simulink model "WaterTankSysControl2024"  (R2024a)
settings: Solver=FixedStepAuto  StartTime=0.0  StopTime=525  FixedStep=0.75  RelTol=1e-3  EnableMultiTasking=on
StopFcn:
  | FileName='SFControlData0.mat';
  | [fPath, fName, fExt] = fileparts(FileName);
  | if isempty(fExt)  % No '.mat' in FileName
  |     fExt     = '.mat';
  |     FileName = fullfile(fPath, [fName, fExt]);
  | end
  | if exist(FileName, 'file')
  |     % Get number of files:
  |     fDir     = dir(fullfile(fPath, [fName, '*', fExt]));
  |     fStr     = lower(sprintf('%s*', fDir.name));
  |     %fNum     = sscanf(fStr, [fName, '%d', fExt, '*']);
  |     digit =  str2double(extract(fStr, digitsPattern));
  |     %newNum = digit + 1;
  |     if isempty(digit)
  |         newNum = 1;
  |     else
  |         newNum = digit + 1;
  |     end
  |     FileName = fullfile(fPath, [fName, sprintf('%d', newNum(end)), fExt]);
  | end
  | save(FileName, 'ScopeData1');
  | clear digit fDir fExt FileName fName fPath fStr newNum fNum
values from neighbouring files (symbols this model uses):
  C_obs = H'    [lab4.m]
  G_obs = G'    [lab4.m]
  Gcl_1 = Gcl_ndb_3    [lab4.m]
  H_obs = C'    [lab4.m]
  K = k1'    [lab4.m]
  L = L_ndb_301    [initialize_control_params.m]    (also in lab4.m)
  u_offset = u_act(1)    [lab4.m]    (also in lanb04.m = 2.5)
  y_offset = mean(y_act(1:i))    [lab4.m]    (also in lanb04.m = mean(y_act(1:i-1)))
undefined symbols (not defined in the file or in its folder): National_Instruments, PCIe
libraries: sldrtlib x4, simulink x1
settings Model: SimulationMode=external  ExtModeTrigDuration=7200  ExtModeArchiveMode=auto  ExtModeArchiveFileName=SysIdenData  ExtModeArchiveDirName=C:\Users\My Project\Documents\MATLAB  ExtModeAutoIncOneShot=on  ExtModeWriteAllDataToWs=on  Creator=My Project  LastModifiedBy=24246
settings SolverCC: AlgebraicLoopSolver=TrustRegion
settings DataIOCC: LimitDataPoints=on  ReturnWorkspaceOutputs=off
settings OptimizationCC: ReuseModelBlockBuffer=off  LifeSpan=inf
settings DebuggingCC: UnconnectedInputMsg=warning  UnconnectedOutputMsg=warning  UnconnectedLineMsg=warning  AllowSymbolicDim=off  SFUnexpectedBacktrackingDiag=warning  SFNoUnconditionalDefaultTransitionDiag=warning  SFExecutionAtInitializationDiag=none  ArithmeticOperatorsInVariantConditions=warning
settings HardwareCC: ProdBitPerLong=64  ProdHWDeviceType=Intel->x86-64 (Linux 64)  TargetBitPerLong=64  TargetBitPerPointer=64  TargetIntDivRoundTo=Zero  TargetEndianess=LittleEndian  TargetWordSize=64  TargetHWDeviceType=Intel->x86-64
settings ModelReferenceCC: EnableRefExpFcnMdlSchedulingChecks=on  PropagateSignalLabelsOutOfModel=off
settings SFSimCC: SimUseLocalCustomCode=off  CustomCodeUndefinedFunction=UseInterfaceOnly
settings RTWCC: Description=Simulink Desktop Real-Time  SystemTargetFile=sldrt.tlc  TemplateMakefile=sldrt.tmf  RTWUseLocalCustomCode=off  RTWCompilerOptimization=on  GPUComputeCapability=3.5
settings CodeAppCC: MaxIdLength=95  StateflowObjectComments=on
settings SimulinkDesktopRealTimeCC: TargetLibSuffix=_sldrt.a  TargetPreCompLibLocation=C:\Program Files\MATLAB\R2024a\toolbox\sldrt\lib\win64  TargetLangStandard=C89/C90 (ANSI)  SupportVariableSizeSignals=off
settings ConfigComp: CovMetricSettings=dw  CovSaveCumulativeToWorkspaceVar=on  CovSaveSingleToWorkspaceVar=on  CovExternalEMLEnable=off

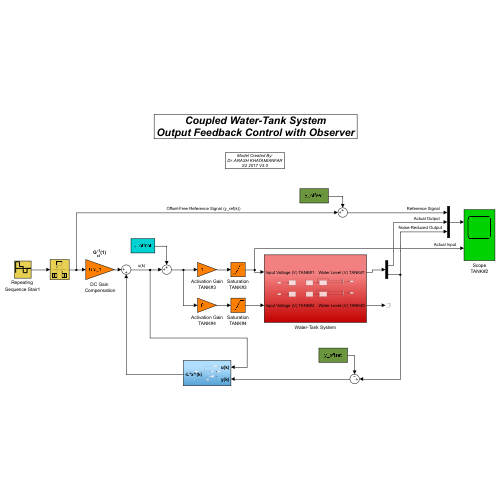
[thumbnail: Simulink's stored preview of the top-level diagram]
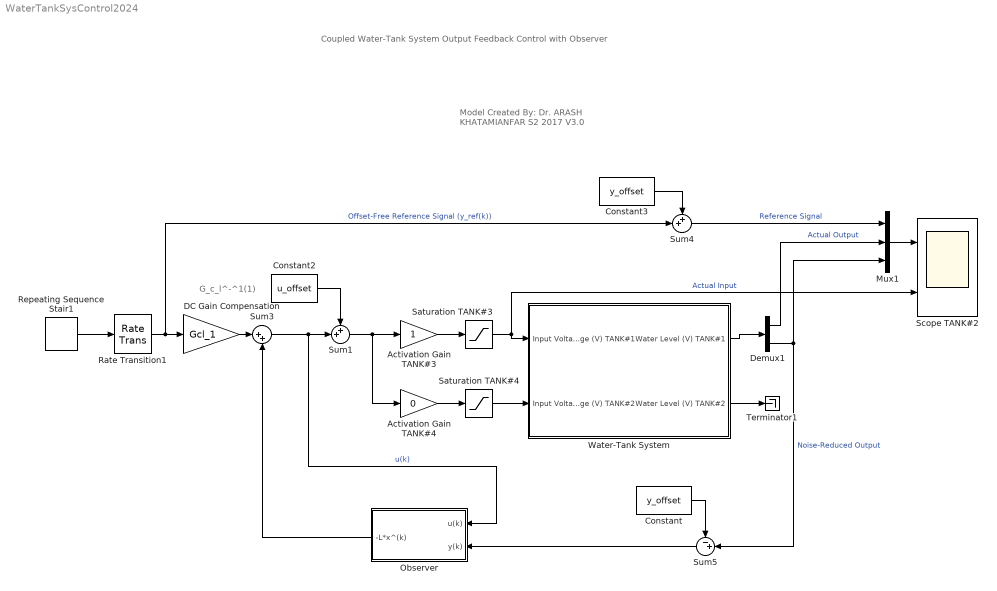
== system WaterTankSysControl2024 ==
  note: Model Created By:
      | Dr. ARASH KHATAMIANFAR
      | S2 2017 V3.0
  note: G_c_l^-^1(1)
  note: Coupled Water-Tank System
      | Output Feedback Control with Observer
  Activation Gain TANK#3 : Gain
  Activation Gain TANK#4 : Gain  Gain=0
  Constant : Constant  Value=y_offset
  Constant2 : Constant  Value=u_offset
  Constant3 : Constant  Value=y_offset
  DC Gain Compensation : Gain  Gain=Gcl_1
  Demux1 : Demux  Outputs=2
  Mux1 : Mux  Inputs=3
  Observer : Subsystem
  Rate Transition1 : RateTransition  OutPortSampleTime=0.75
  Repeating Sequence Stair1 : simulink/Sources/Repeating Sequence Stair  OutValues=[0.7 0.2 -0.5 0].'  tsamp=140*0.75  OutMin=[]  OutMax=[]  OutDataTypeStr=double  OutputDataTypeScalingMode=double  OutDataType=fixdt(0,8)  ConRadixGroup=Best Precision: Vector-wise  OutScaling=2^-12
  Saturation TANK#3 : Saturate  UpperLimit=3.0  LowerLimit=1.5
  Saturation TANK#4 : Saturate  UpperLimit=5  LowerLimit=0
  Scope TANK#2 : Scope  NumInputPorts=2
  Sum1 : Sum  Inputs=++|
  Sum3 : Sum  Inputs=|++
  Sum4 : Sum  Inputs=++|
  Sum5 : Sum  Inputs=-+|
  Terminator1 : Terminator
  Water-Tank System : Subsystem
  wires:
  Demux1/2 -> Sum5/2, Mux1/3  "Noise-Reduced Output"
  Demux1/1 -> Mux1/2  "Actual Output"
  Saturation TANK#3/1 -> Water-Tank System/1(Input Voltage (V) TANK#1), Scope TANK#2/2  "Actual Input"
  DC Gain Compensation/1 -> Sum3/1
  Repeating Sequence Stair1/1 -> Rate Transition1/1
  Sum4/1 -> Mux1/1  "Reference Signal"
  Water-Tank System/1(Water Level (V) TANK#1) -> Demux1/1
  Rate Transition1/1 -> Sum4/2, DC Gain Compensation/1  "Offset-Free Reference Signal (y_ref(k))"
  Water-Tank System/2(Water Level (V) TANK#2) -> Terminator1/1
  Constant/1 -> Sum5/1
  Sum1/1 -> Activation Gain TANK#4/1, Activation Gain TANK#3/1
  Saturation TANK#4/1 -> Water-Tank System/2(Input Voltage (V) TANK#2)
  Activation Gain TANK#3/1 -> Saturation TANK#3/1
  Mux1/1 -> Scope TANK#2/1
  Sum3/1 -> Observer/1(u(k)), Sum1/2  "u(k)"
  Activation Gain TANK#4/1 -> Saturation TANK#4/1
  Constant3/1 -> Sum4/1
  Observer/1(-L*x^(k)) -> Sum3/2
  Sum5/1 -> Observer/2(y(k))
  Constant2/1 -> Sum1/1

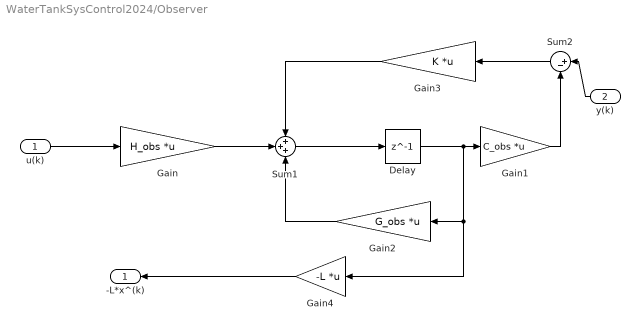
== system WaterTankSysControl2024/Observer ==
  u(k) : Inport
  y(k) : Inport  Port=2
  Delay : Delay  DelayLength=1  InitialCondition=[0;0]  SampleTime=0.75
  Gain : Gain  Gain=H_obs  Multiplication=Matrix(K*u)
  Gain1 : Gain  Gain=C_obs  Multiplication=Matrix(K*u)
  Gain2 : Gain  Gain=G_obs  Multiplication=Matrix(K*u)
  Gain3 : Gain  Gain=K  Multiplication=Matrix(K*u)
  Gain4 : Gain  Gain=-L  Multiplication=Matrix(K*u)
  Sum1 : Sum  Inputs=+++
  Sum2 : Sum  Inputs=|+-
  -L*x^(k) : Outport  VectorParamsAs1DForOutWhenUnconnected=off
  wires:
  Delay/1 -> Gain1/1, Gain4/1, Gain2/1
  Sum2/1 -> Gain3/1
  Sum1/1 -> Delay/1
  Gain/1 -> Sum1/2
  Gain1/1 -> Sum2/2
  Gain2/1 -> Sum1/3
  Gain3/1 -> Sum1/1
  y(k)/1 -> Sum2/1
  u(k)/1 -> Gain/1
  Gain4/1 -> -L*x^(k)/1

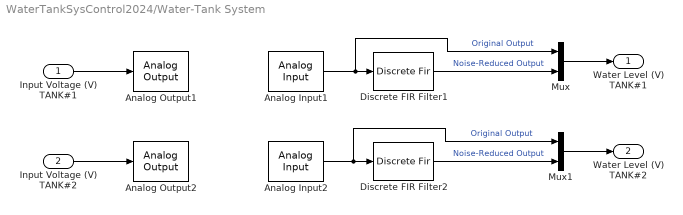
== system WaterTankSysControl2024/Water-Tank System ==
  Input Voltage (V) TANK#1 : Inport
  Input Voltage (V) TANK#2 : Inport  Port=2
  Analog Input1 : sldrtlib/Analog Input  SampleTime=0.75  MaxMissedTicks=10  ShowMissedTicks=off  YieldWhenWaiting=off  DrvName=National_Instruments/PCIe-6351  DrvAddress=4294967295  DrvOptions=[0 0 0 0 0 0 0]  Channels=1  RangeMode=1  VoltRange=1  DataType=1
      settings: AttributesFormatString=National Instruments\nPCIe-6351 [auto]
  Analog Input2 : sldrtlib/Analog Input  SampleTime=0.75  MaxMissedTicks=10  ShowMissedTicks=off  YieldWhenWaiting=off  DrvName=National_Instruments/PCIe-6351  DrvAddress=4294967295  DrvOptions=[0 0 0 0 0 0 0]  Channels=2  RangeMode=1  VoltRange=1  DataType=1
      settings: AttributesFormatString=National Instruments\nPCIe-6351 [auto]
  Analog Output1 : sldrtlib/Analog Output  SampleTime=0.75  MaxMissedTicks=10  ShowMissedTicks=off  YieldWhenWaiting=off  DrvName=National_Instruments/PCIe-6351  DrvAddress=4294967295  DrvOptions=[0 0 0 0 0 0 0]  Channels=1  RangeMode=1  VoltRange=1  InitialValue=0  FinalValue=0
      settings: AttributesFormatString=National Instruments\nPCIe-6351 [auto]
  Analog Output2 : sldrtlib/Analog Output  SampleTime=0.75  MaxMissedTicks=10  ShowMissedTicks=off  YieldWhenWaiting=off  DrvName=National_Instruments/PCIe-6351  DrvAddress=4294967295  DrvOptions=[0 0 0 0 0 0 0]  Channels=2  RangeMode=1  VoltRange=1  InitialValue=0  FinalValue=0
      settings: AttributesFormatString=National Instruments\nPCIe-6351 [auto]
  Discrete FIR Filter1 : DiscreteFir  Coefficients=[0.2 0.2 0.2 0.2 0.2]  SampleTime=0.75
  Discrete FIR Filter2 : DiscreteFir  Coefficients=[0.2 0.2 0.2 0.2 0.2]  SampleTime=0.75
  Mux : Mux  Inputs=2
  Mux1 : Mux  Inputs=2
  Water Level (V) TANK#1 : Outport
  Water Level (V) TANK#2 : Outport  Port=2
  wires:
  Analog Input1/1 -> Mux/1, Discrete FIR Filter1/1  "Original Output"
  Input Voltage (V) TANK#1/1 -> Analog Output1/1
  Discrete FIR Filter1/1 -> Mux/2  "Noise-Reduced Output"
  Mux/1 -> Water Level (V) TANK#1/1
  Analog Input2/1 -> Mux1/1, Discrete FIR Filter2/1  "Original Output"
  Input Voltage (V) TANK#2/1 -> Analog Output2/1
  Discrete FIR Filter2/1 -> Mux1/2  "Noise-Reduced Output"
  Mux1/1 -> Water Level (V) TANK#2/1
